simulink model "root_model"  (R2025b)
settings: Solver=VariableStepAuto  StartTime=0.0  StopTime=200  RelTol=1e-3
model workspace (MAT data in the model file):
  body_len = 0.435
  body_mass = 1.206
  body_radius = 0.035
  g = 9.81
  inertia_tensor = Simulink.Parameter
  inertia_tensor.Value = [0.01938645  0  0; 0  0.01938645  0; 0  0  0.000738675]
  inertia_tensor.Complexity = 'real'
  inertia_tensor.Dimensions = [3 3]
  inertia_tensor.Description = 'https://en.wikipedia.org/wiki/List_of_moments_of_inertia#List_of_3D_inertia'
  inertia_tensor.DataType = 'auto'
  lever_arm = 0.242
  max_rps = 167
  out = Simulink.SimulationOutput
  out.Data.tout = [0 3.15544362088e-30 3.33352544411e-06 2.00011526647e-05 0.000103339288767 0.000520029969281 0.00260348337185 0.0130207503847 0.0651070854489 0.1 0.159208772587 0.2 ... (2663 elements, 2663x1)]
  out.Metadata = Simulink.SimulationMetadata
  out.Metadata.ModelInfo.ModelName = 'root_model'
  out.Metadata.ModelInfo.ModelVersion = '1.8'
  out.Metadata.ModelInfo.ModelFilePath = 'C:\Users\Josh\Documents\MTU\Involvement\AERE\simulink-testing\mpc-6dof-model\root_model.slx'
  out.Metadata.ModelInfo.UserID = 'Josh'
  out.Metadata.ModelInfo.MachineName = 'DESKTOP-E2GQ9U1'
  out.Metadata.ModelInfo.Platform = 'PCWIN64'
  out.Metadata.ModelInfo.ModelStructuralChecksum = [3232016487; 973311862; 3022833271; 3161490746]
  out.Metadata.ModelInfo.SimulationMode = 'normal'
  out.Metadata.ModelInfo.StartTime = 0
  out.Metadata.ModelInfo.StopTime = 10
  out.Metadata.ModelInfo.SolverInfo.Type = 'Variable-Step'
  out.Metadata.ModelInfo.SolverInfo.Solver = 'ode45'
  out.Metadata.ModelInfo.SolverInfo.MaxStepSize = 0.1
  out.Metadata.ModelInfo.SimulinkVersion.Name = 'Simulink'
  out.Metadata.ModelInfo.SimulinkVersion.Version = '25.2'
  out.Metadata.ModelInfo.SimulinkVersion.Release = '(R2025b)'
  out.Metadata.ModelInfo.SimulinkVersion.Date = '28-Jul-2025'
  out.Metadata.ModelInfo.LoggingInfo.LoggingToFile = 'off'
  out.Metadata.TimingInfo.WallClockTimestampStart = '2026-04-01 21:49:39'
  out.Metadata.TimingInfo.WallClockTimestampStop = '2026-04-01 21:49:46'
  out.Metadata.TimingInfo.InitializationElapsedWallTime = 0.363943
  out.Metadata.TimingInfo.ExecutionElapsedWallTime = 6.470538
  out.Metadata.TimingInfo.TerminationElapsedWallTime = 0.0036556
  out.Metadata.TimingInfo.TotalElapsedWallTime = 6.8381366
  out.Metadata.TimingInfo.ProfilerData = 'Profiler is not enabled'
  out.Metadata.ExecutionInfo.StopEvent = 'ReachedStopTime'
  out.Metadata.ExecutionInfo.StopEventSource = []
  out.Metadata.ExecutionInfo.StopEventDescription = 'Reached stop time of 10'
  out.Metadata.ExecutionInfo.ErrorDiagnostic = []
  out.Metadata.ExecutionInfo.WarningDiagnostics = struct([])
  out.Metadata.AppInfo = struct()
  prop_const = 0.0005967898212
  w_mv = [0.1 0.1 0.1]
  w_mvr = [0.1 0.5 0.5]
  w_ov = [1 1 1 0.1 0.1 0.1 0 0 0 0 0.1 0.1 0.1]
values from neighbouring files (symbols this model uses):
  inertia_tensor = eye(3)    [vehicle_mpc.m]
libraries: checkpacklib x5, mpclib x1
settings Model: Creator=Josh  LastModifiedBy=Josh Fernandez
settings DebuggingCC: SignalInfNanChecking=error

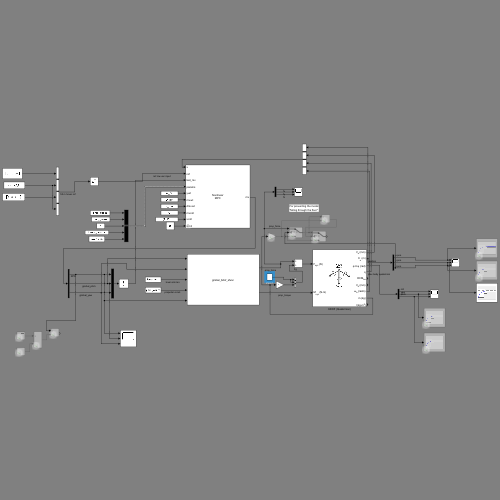
[thumbnail: Simulink's stored preview of the top-level diagram]
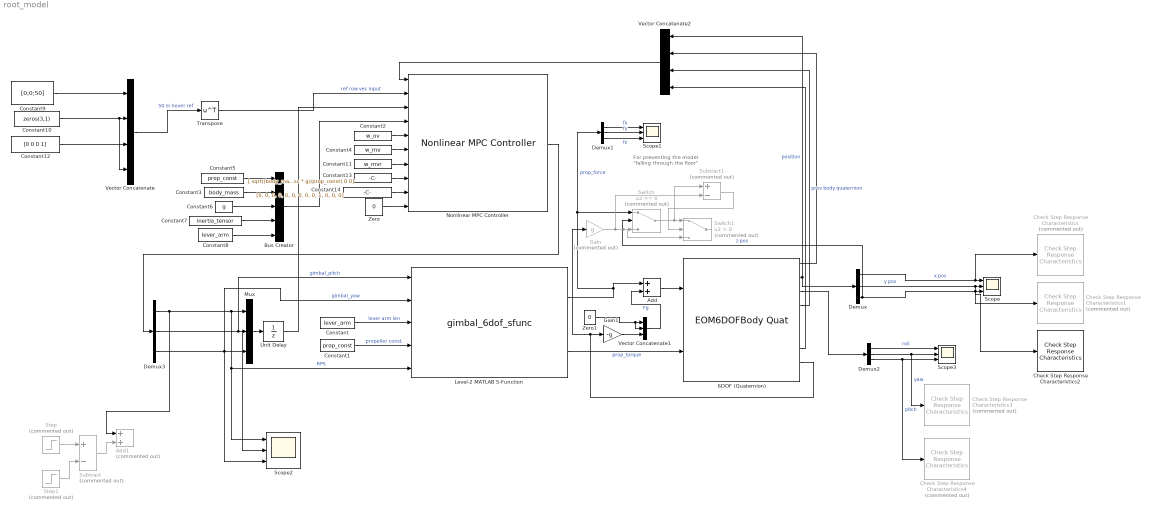
== system root_model ==
  note: For preventing the model
      | "falling through the floor"
  6DOF (Quaternion) : EOM6DOFBodyQuat  mass_0=body_mass  inertia=inertia_tensor  mass_flag=on
  Add : Sum
  Add1 : Sum  Commented=on
  Bus Creator : BusCreator  Inputs=5  OutDataTypeStr=Bus: mpc_params_bus  NonVirtualBus=on
      settings: InheritFromInputs=off
  Check Step Response Characteristics{,1,3..4} (4 alike) : checkpacklib/Check Step Response  Characteristics  Commented=on  InstantiateOnLoad=on  enabled=on  stopWhenAssertionFail=off  export=off  ViewDlgPos=[]  OpenViewOnLoad=off  LaunchViewOnOpen=off  TimeUnits=seconds  EnableStepResponseBound=on  InitialValue=0  FinalValue=0  StepTime=0  RiseTime=5  PercentRise=80  SettlingTime=7  PercentSettling=1  PercentOvershoot=10  PercentUndershoot=1
      settings: LibrarySourceBlock=|
      | sdolib/Model Verification/Check Step Response
      | Characteristics
  Check Step Response Characteristics2 : checkpacklib/Check Step Response  Characteristics  InstantiateOnLoad=on  enabled=on  stopWhenAssertionFail=off  export=off  ViewDlgPos=[100 200 510 390]  OpenViewOnLoad=off  LaunchViewOnOpen=off  TimeUnits=seconds  EnableStepResponseBound=on  InitialValue=0  FinalValue=50  StepTime=0  RiseTime=20  PercentRise=80  SettlingTime=30  PercentSettling=1  PercentOvershoot=10  PercentUndershoot=1
      settings: LibrarySourceBlock=|
      | sdolib/Model Verification/Check Step Response
      | Characteristics
  Constant : Constant  Value=lever_arm
  Constant1 : Constant  Value=prop_const
  Constant10 : Constant  Value=zeros(3,1)
  Constant11 : Constant  Value=w_mvr  VectorParams1D=off
  Constant12 : Constant  Value=[0 0 0 1]
  Constant13 : Constant  Value=[ sqrt((body_mass * g)/prop_const) 0 0]  VectorParams1D=off
  Constant14 : Constant  Value=[0, 0, 0, 0, 0, 0, 0, 0, 0, 1, 0, 0, 0]  VectorParams1D=off
  Constant2 : Constant  Value=w_ov  VectorParams1D=off
  Constant3 : Constant  Value=body_mass
  Constant4 : Constant  Value=w_mv  VectorParams1D=off
  Constant5 : Constant  Value=prop_const
  Constant6 : Constant  Value=g
  Constant7 : Constant  Value=inertia_tensor
  Constant8 : Constant  Value=lever_arm
  Constant9 : Constant  Value=[0;0;50]
  Demux{,1..3} (4 alike) : Demux  Outputs=3
  Gain : Gain  Commented=on  Gain=g
  Gain1 : Gain  Gain=-g
  Level-2 MATLAB S-Function : M-S-Function  FunctionName=gimbal_6dof_sfunc
  Mux : Mux  Inputs=3
  Nonlinear MPC Controller : mpclib/Nonlinear MPC Controller  nlmpcobj=mpc_obj  UseObjectTs=on  UseMEX=off  md_enabled=off  mvtarget_enabled=off  param_enabled=on  cost_enabled=off  mvseq_enabled=off  stateseq_enabled=off  ovseq_enabled=off  slack_enabled=off  status_enabled=off  ov_min=off  ov_max=off  mv_min=off  mv_max=off  mvrate_min=off  mvrate_max=off  state_min=off  state_max=off  ov_weight=on  mv_weight=on  mvrate_weight=on  ecr_weight=off  nlp_initialize=on
  Scope{,1..3} (4 alike) : Scope  NumInputPorts=3
      Scope settings: ActiveDisplayYMinimum=-1794.9066759996349  ActiveDisplayYMaximum=2241.5668757479152
      Scope1 settings: ActiveDisplayYMinimum=4.29292633197872  ActiveDisplayYMaximum=72.484649474443529
      Scope2 settings: ActiveDisplayYMinimum=-0.017983278944692226  ActiveDisplayYMaximum=0.017982670853515178  DataLoggingVariableName=ScopeData2
      Scope3 settings: ActiveDisplayYMinimum=-4.8883170553412256  ActiveDisplayYMaximum=4.9767170632167073  DataLoggingVariableName=ScopeData3
  Step : Step  Commented=on  After=50  SampleTime=0
  Step1 : Step  Commented=on  Time=2  After=50  SampleTime=0
  Subtract : Sum  Commented=on  Inputs=+-
  Subtract1 : Sum  Commented=on  Inputs=+-
  Switch : Switch  Commented=on  SaturateOnIntegerOverflow=off  InputSameDT=off
  Switch1 : Switch  Commented=on  Criteria=u2 > Threshold  SaturateOnIntegerOverflow=off  InputSameDT=off
  Transpose : Math  Operator=transpose
  Unit Delay : UnitDelay  SampleTime=-1  HasFrameUpgradeWarning=on
  Vector Concatenate : Concatenate  NumInputs=4
  Vector Concatenate1 : Concatenate  NumInputs=3
  Vector Concatenate2 : Concatenate  NumInputs=4
  Zero : Constant  Value=0  OutDataTypeStr=Inherit: Inherit via back propagation
  Zero1 : Constant  Value=0  OutDataTypeStr=Inherit: Inherit via back propagation
  wires:
  Level-2 MATLAB S-Function/1 -> Add/1, Demux1/1, Switch/1  "prop_force"
  Level-2 MATLAB S-Function/2 -> 6DOF (Quaternion)/2  "prop_torque"
  Constant/1 -> Level-2 MATLAB S-Function/3  "lever arm len"
  Constant1/1 -> Level-2 MATLAB S-Function/4  "propeller const."
  6DOF (Quaternion)/2 -> Demux/1, Vector Concatenate2/1  "position"
  6DOF (Quaternion)/3 -> Demux2/1
  Demux2/2 -> Check Step Response Characteristics3/1, Scope3/2  "yaw"
  Demux2/3 -> Scope3/3, Check Step Response Characteristics4/1  "pitch"
  Demux2/1 -> Scope3/1  "roll"
  Demux/2 -> Check Step Response Characteristics1/1, Scope/2  "y pos"
  Demux/3 -> Switch/2, Check Step Response Characteristics2/1, Scope/3  "z pos"
  Demux/1 -> Check Step Response Characteristics/1, Scope/1  "x pos"
  Demux1/1 -> Scope1/1  "fx"
  Demux1/2 -> Scope1/2  "fy"
  Demux1/3 -> Scope1/3  "fz"
  Constant3/1 -> Bus Creator/2
  Add/1 -> 6DOF (Quaternion)/1
  Gain1/1 -> Vector Concatenate1/3
  Zero1/1 -> Vector Concatenate1/2, Vector Concatenate1/1
  Vector Concatenate1/1 -> Add/2  "Fg"
  Constant5/1 -> Bus Creator/1
  Constant6/1 -> Bus Creator/3
  Bus Creator/1 -> Nonlinear MPC Controller/4
  Constant9/1 -> Vector Concatenate/1
  Constant10/1 -> Vector Concatenate/4, Vector Concatenate/2
  Constant12/1 -> Vector Concatenate/3
  Vector Concatenate/1 -> Transpose/1  "50 m hover ref"
  6DOF (Quaternion)/1 -> Vector Concatenate2/2
  6DOF (Quaternion)/4 -> Vector Concatenate2/3  "prev body quaternion"
  6DOF (Quaternion)/7 -> Vector Concatenate2/4
  Transpose/1 -> Nonlinear MPC Controller/2  "ref row vec input"
  Vector Concatenate2/1 -> Nonlinear MPC Controller/1
  Constant8/1 -> Bus Creator/5
  Constant7/1 -> Bus Creator/4
  Nonlinear MPC Controller/1 -> Demux3/1
  Demux3/3 -> Mux/3, Level-2 MATLAB S-Function/2, Scope2/3  "gimbal_yaw"
  Demux3/2 -> Scope2/2, Level-2 MATLAB S-Function/1, Mux/2  "gimbal_pitch"
  Demux3/1 -> Mux/1, Level-2 MATLAB S-Function/5, Scope2/1, Add1/1  "RPS"
  Mux/1 -> Unit Delay/1
  Unit Delay/1 -> Nonlinear MPC Controller/3
  Step/1 -> Subtract/1
  Subtract/1 -> Add1/2
  Step1/1 -> Subtract/2
  6DOF (Quaternion)/8 -> Gain/1, Gain1/1
  Constant2/1 -> Nonlinear MPC Controller/5
  Constant4/1 -> Nonlinear MPC Controller/6
  Constant11/1 -> Nonlinear MPC Controller/7
  Gain/1 -> Switch1/3, Switch/3, Subtract1/2
  Switch/1 -> Subtract1/1, Switch1/1
  Subtract1/1 -> Switch1/2
  Constant13/1 -> Nonlinear MPC Controller/8
  Constant14/1 -> Nonlinear MPC Controller/9
  Zero/1 -> Nonlinear MPC Controller/10
